simulink model "Pendelum_Model_2016"  (R2016a)
settings: Solver=VariableStepAuto  SolverMode=SingleTasking  StartTime=0.0  StopTime=Sim_Time  MaxStep=0.01  RelTol=1e-3
values from neighbouring files (symbols this model uses):
  b = 0.1    [PendelumScript.m]
  g = 9.81    [PendelumScript.m]
  I = 0.0027    [PendelumScript.m]
  Kd = 25    [PendelumScript.m]
  Ki = 1    [PendelumScript.m]
  Kp = 120    [PendelumScript.m]
  l = 0.178    [PendelumScript.m]
  m = 0.065    [PendelumScript.m]
  M = 0.6    [PendelumScript.m]
libraries: simulink x1
settings Model: Creator=k1447508  LastModifiedBy=Funsho
settings SolverCC: AlgebraicLoopSolver=LineSearch
settings DebuggingCC: SFUnexpectedBacktrackingDiag=error  SFNoUnconditionalDefaultTransitionDiag=error
settings SFSimCC: SimUseLocalCustomCode=on
settings RTWCC: RTWUseLocalCustomCode=on
settings GRTTargetCC: TargetLangStandard=C99 (ISO)  GeneratePreprocessorConditionals=Use local settings
settings ConfigComp: CovMetricSettings=dwe  CovHtmlReporting=off  CovSaveCumulativeToWorkspaceVar=off  CovSaveSingleToWorkspaceVar=off  CovExternalEMLEnable=on

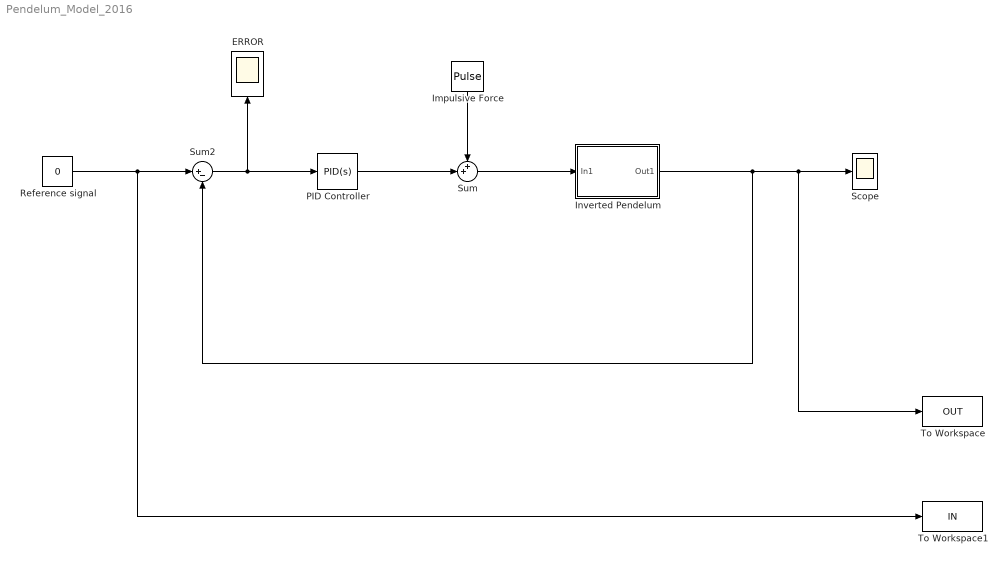
== system Pendelum_Model_2016 ==
  " Impulsive Force" : DiscretePulseGenerator  PulseType=Time based  Amplitude=1000  Period=10  PulseWidth=0.01
  ERROR : Scope
  Inverted Pendelum : Subsystem
  PID Controller : simulink/Continuous/PID Controller  Controller=PID  TimeDomain=Continuous-time  SampleTime=-1  IntegratorMethod=Forward Euler  FilterMethod=Forward Euler  Form=Parallel  UseFilter=on  ControllerParametersSource=internal  P=Kp  I=Ki  D=Kd  N=100  InitialConditionSource=internal  InitialConditionForIntegrator=0  InitialConditionForFilter=0  ExternalReset=none  LimitOutput=off  UpperSaturationLimit=inf  LowerSaturationLimit=-inf  LinearizeAsGain=on  AntiWindupMode=none  Kb=1  TrackingMode=off  Kt=1  PParamMin=[]  PParamMax=[]  IParamMin=[]  IParamMax=[]  DParamMin=[]  DParamMax=[]  NParamMin=[]  NParamMax=[]  KbParamMin=[]  KbParamMax=[]  KtParamMin=[]  KtParamMax=[]  POutMin=[]  POutMax=[]  IOutMin=[]  IOutMax=[]  DOutMin=[]  DOutMax=[]  NOutMin=[]  NOutMax=[]  KbOutMin=[]  KbOutMax=[]  KtOutMin=[]  KtOutMax=[]  IntegratorOutMin=[]  IntegratorOutMax=[]  FilterOutMin=[]  FilterOutMax=[]  SumOutMin=[]  SumOutMax=[]  SumI1OutMin=[]  SumI1OutMax=[]  SumI2OutMin=[]  SumI2OutMax=[]  SumI3OutMin=[]  SumI3OutMax=[]  SumDOutMin=[]  SumDOutMax=[]  SaturationOutMin=[]  SaturationOutMax=[]  IntegratorContinuousStateAttributes=''  IntegratorStateMustResolveToSignalObject=off  IntegratorRTWStateStorageClass=Auto  FilterContinuousStateAttributes=''  FilterStateMustResolveToSignalObject=off  FilterRTWStateStorageClass=Auto  DifferentiatorICPrevScaledInput=0  DifferentiatorOutMin=[]  DifferentiatorOutMax=[]
  Reference signal : Constant  Value=0
  Scope : Scope
  Sum : Sum  Inputs=++|
  Sum2 : Sum  Inputs=|+-
  To Workspace : ToWorkspace  VariableName=OUT  SaveFormat=Timeseries  SampleTime=-1
  To Workspace1 : ToWorkspace  VariableName=IN  SaveFormat=Timeseries  SampleTime=-1
  wires:
  Reference signal/1 -> To Workspace1/1, Sum2/1
  Sum2/1 -> PID Controller/1, ERROR/1
  Inverted Pendelum/1(Out1) -> To Workspace/1, Scope/1, Sum2/2
  " Impulsive Force"/1 -> Sum/1
  PID Controller/1 -> Sum/2
  Sum/1 -> Inverted Pendelum/1(In1)

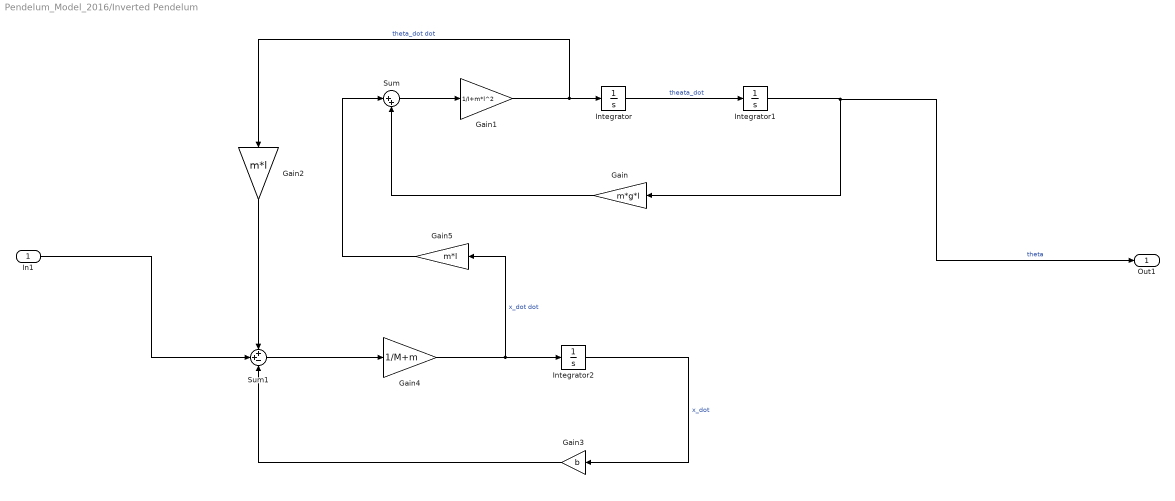
== system Pendelum_Model_2016/Inverted Pendelum ==
  In1 : Inport
  Gain : Gain  Gain=m*g*l
  Gain1 : Gain  Gain=1/I+m*l^2
  Gain2 : Gain  Gain=m*l
  Gain3 : Gain  Gain=b
  Gain4 : Gain  Gain=1/M+m
  Gain5 : Gain  Gain=m*l
  Integrator : Integrator
  Integrator1 : Integrator
  Integrator2 : Integrator
  Sum : Sum  Inputs=|++
  Sum1 : Sum  Inputs=++-
  Out1 : Outport
  wires:
  In1/1 -> Sum1/2
  Gain3/1 -> Sum1/3
  Gain5/1 -> Sum/1
  Gain/1 -> Sum/2
  Gain2/1 -> Sum1/1
  Gain4/1 -> Gain5/1, Integrator2/1  "x_dot dot"
  Sum1/1 -> Gain4/1
  Sum/1 -> Gain1/1
  Integrator2/1 -> Gain3/1  "x_dot"
  Gain1/1 -> Gain2/1, Integrator/1  "theta_dot dot"
  Integrator/1 -> Integrator1/1  "theata_dot"
  Integrator1/1 -> Out1/1, Gain/1  "theta"
